simulink model "simu_acc"  (R2019b)
settings: Solver=VariableStepAuto  StartTime=0.0  StopTime=200.0  RelTol=1e-3
values from neighbouring files (symbols this model uses):
  d_0 = 150    [parametros.m]
  d_ref = 50    [parametros.m]
  delta_d_ref = 0    [parametros.m]
  delta_theta = 0    [parametros.m]
  delta_u_ref = 0    [parametros.m]
  delta_uw = 0    [parametros.m]
  delta_vl = -5    [parametros.m]
  K = 1/(rho*Cd*A*(V0 + VW0))    [modelo_lin.m]
  Kd_pos = 0    [parametros.m]
  Kd_vel = 0    [parametros.m]
  Ki_pos = 0    [parametros.m]
  Ki_vel = 5    [parametros.m]
  Kp_pos = 0.08    [parametros.m]
  Kp_vel = 100    [parametros.m]
  pend_vl = 1    [parametros.m]
  t_pert = 150    [parametros.m]
  t_ref = 20    [parametros.m]
  t_vl = 150    [parametros.m]
  tau = m/(rho*Cd*A*(V0 + VW0))    [modelo_lin.m]
  theta = in(3)    [dinamica.m]    (also in parametros.m = 0)
  u_ini = 20    [parametros.m]
  u_ref = 20    [parametros.m]
  uw = in(2)    [dinamica.m]    (also in parametros.m = 20)
  vl = 18    [parametros.m]
  wc_filt_vel = 5    [parametros.m]
libraries: simulink x6
settings Model: Creator=isidro  LastModifiedBy=isidro

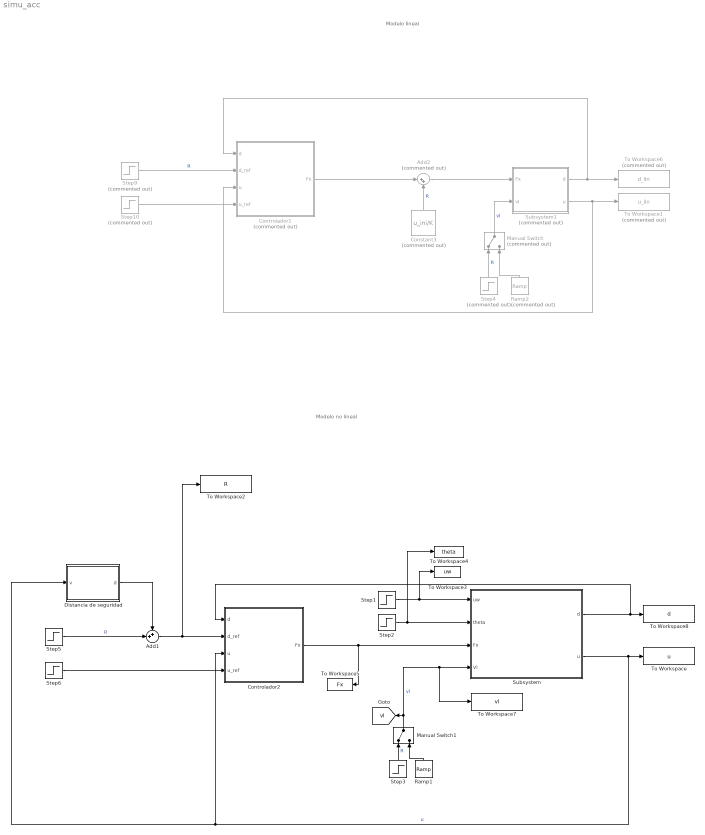
== system simu_acc ==
  note: Modelo no lineal
  note: Modelo lineal
  Add1 : Sum  Inputs=++|
  Add2 : Sum  Commented=on  Inputs=|++
  Constant3 : Constant  Commented=on  Value=u_ini/K  SampleTime=0
  Controlador1 : Subsystem  Commented=on
  Controlador2 : Subsystem
  Distancia de seguridad : Subsystem
  Manual Switch : ManualSwitch  Commented=on
  Manual Switch1 : ManualSwitch
  Ramp1 : simulink/Sources/Ramp  slope=pend_vl  start=t_vl  InitialOutput=vl
  Ramp2 : simulink/Sources/Ramp  Commented=on  slope=pend_vl  start=t_vl  InitialOutput=vl
  Step1 : Step  Time=t_pert  Before=uw  After=uw+delta_uw  SampleTime=0
  Step10 : Step  Commented=on  Time=t_ref  Before=u_ref  After=u_ref + delta_u_ref  SampleTime=0
  Step2 : Step  Time=t_pert  Before=theta  After=theta+delta_theta  SampleTime=0
  Step3 : Step  Time=t_vl  Before=vl  After=delta_vl+vl  SampleTime=0
  Step4 : Step  Commented=on  Time=t_vl  Before=vl  After=delta_vl+vl  SampleTime=0
  Step5 : Step  Time=t_ref  Before=d_ref  After=d_ref + delta_d_ref  SampleTime=0
  Step6 : Step  Time=t_ref  Before=u_ref  After=u_ref + delta_u_ref  SampleTime=0
  Step9 : Step  Commented=on  Time=t_ref  Before=d_ref  After=d_ref + delta_d_ref  SampleTime=0
  Subsystem : Subsystem
  Subsystem1 : Subsystem  Commented=on
  To Workspace : ToWorkspace  VariableName=u  SaveFormat=Timeseries  SampleTime=-1
  To Workspace1 : ToWorkspace  Commented=on  VariableName=u_lin  SaveFormat=Timeseries  SampleTime=-1
  To Workspace2 : ToWorkspace  VariableName=R  SaveFormat=Timeseries  SampleTime=-1
  To Workspace3 : ToWorkspace  VariableName=uw  SaveFormat=Timeseries  SampleTime=-1
  To Workspace4 : ToWorkspace  VariableName=theta  SaveFormat=Timeseries  SampleTime=-1
  To Workspace5 : ToWorkspace  VariableName=Fx  SaveFormat=Timeseries  SampleTime=-1
  To Workspace6 : ToWorkspace  Commented=on  VariableName=d_lin  SaveFormat=Timeseries  SampleTime=-1
  To Workspace7 : ToWorkspace  VariableName=vl  SaveFormat=Timeseries  SampleTime=-1
  To Workspace8 : ToWorkspace  VariableName=d  SaveFormat=Timeseries  SampleTime=-1
  tag scope: vl=global
  wires:
  Subsystem/2(u) -> Controlador2/3(u), Distancia de seguridad/1(v), To Workspace/1  "u"
  Step1/1 -> To Workspace3/1, Subsystem/1(uw)
  Step2/1 -> To Workspace4/1, Subsystem/2(theta)
  Step4/1 -> Manual Switch/1  "R"
  Ramp2/1 -> Manual Switch/2
  Manual Switch/1 -> Subsystem1/2(vl)  "vl"
  Subsystem1/2(u) -> Controlador1/3(u), To Workspace1/1
  Subsystem1/1(d) -> Controlador1/1(d), To Workspace6/1
  Manual Switch1/1 -> [vl], To Workspace7/1, Subsystem/4(Vl)  "vl"
  Ramp1/1 -> Manual Switch1/2
  Step3/1 -> Manual Switch1/1  "R"
  Subsystem/1(d) -> Controlador2/1(d), To Workspace8/1
  Constant3/1 -> Add2/2  "R"
  Add2/1 -> Subsystem1/1(Fx)
  Step6/1 -> Controlador2/4(u_ref)
  Controlador2/1(Fx) -> To Workspace5/1, Subsystem/3(Fx)
  Step10/1 -> Controlador1/4(u_ref)
  Controlador1/1(Fx) -> Add2/1
  Step9/1 -> Controlador1/2(d_ref)  "R"
  Distancia de seguridad/1(d) -> Add1/1
  Step5/1 -> Add1/2  "R"
  Add1/1 -> To Workspace2/1, Controlador2/2(d_ref)

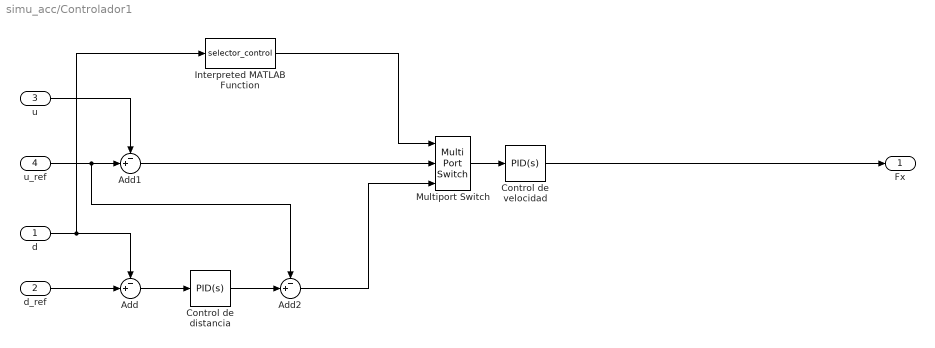
== system simu_acc/Controlador1 ==
  d : Inport
  d_ref : Inport  Port=2
  u : Inport  Port=3
  u_ref : Inport  Port=4
  Add : Sum  Inputs=-+|
  Add1 : Sum  Inputs=-+|
  Add2 : Sum  Inputs=-+|
  Control de distancia : simulink/Continuous/PID Controller  Controller=PID  Form=Parallel  TimeDomain=Continuous-time  SampleTime=-1  IntegratorMethod=Forward Euler  FilterMethod=Forward Euler  ControllerParametersSource=internal  P=Kp_pos  I=Ki_pos  D=Kd_pos  UseFilter=on  N=100  TunerSelectOption=Transfer Function Based (PID Tuner App)  InitialConditionSource=internal  InitialConditionForIntegrator=0  InitialConditionForFilter=0  DifferentiatorICPrevScaledInput=0  ExternalReset=none  TrackingMode=off  Kt=1  LimitOutput=off  UpperSaturationLimit=inf  LowerSaturationLimit=-inf  LinearizeAsGain=on  AntiWindupMode=none  Kb=1  POutMin=[]  POutMax=[]  IOutMin=[]  IOutMax=[]  DOutMin=[]  DOutMax=[]  NOutMin=[]  NOutMax=[]  SumOutMin=[]  SumOutMax=[]  SaturationOutMin=[]  SaturationOutMax=[]  PParamMin=[]  PParamMax=[]  IParamMin=[]  IParamMax=[]  DParamMin=[]  DParamMax=[]  NParamMin=[]  NParamMax=[]  KbParamMin=[]  KbParamMax=[]  KtParamMin=[]  KtParamMax=[]  KbOutMin=[]  KbOutMax=[]  KtOutMin=[]  KtOutMax=[]  IntegratorOutMin=[]  IntegratorOutMax=[]  FilterOutMin=[]  FilterOutMax=[]  SumI1OutMin=[]  SumI1OutMax=[]  SumI2OutMin=[]  SumI2OutMax=[]  SumI3OutMin=[]  SumI3OutMax=[]  SumI4OutMin=[]  SumI4OutMax=[]  SumDOutMin=[]  SumDOutMax=[]  DifferentiatorOutMin=[]  DifferentiatorOutMax=[]  FilterDiffOutCoefMin=[]  FilterDiffOutCoefMax=[]  ReciprocalOutMin=[]  ReciprocalOutMax=[]  SumDenOutMin=[]  SumDenOutMax=[]  SumNumOutMin=[]  SumNumOutMax=[]  DivideOutMin=[]  DivideOutMax=[]  IntegratorContinuousStateAttributes=''  IntegratorStateMustResolveToSignalObject=off  IntegratorRTWStateStorageClass=Auto  FilterContinuousStateAttributes=''  FilterStateMustResolveToSignalObject=off  FilterRTWStateStorageClass=Auto  ParallelPVariant=InternalParameters  IdealPVariant=Disabled  IVariant=InternalParameters  DVariant=InternalParameters  IntegratorVariant=Continuous  SatVariant=Disabled  AWVariant=Passthrough  PCopyVariant=Disabled  TRVariant=Disabled  FdbkBlocksVariant=Forward  IdealPFdbkVariant=Disabled  SatFdbkVariant=Disabled  DerivativeFilterVariant=ContFilter  NVariant=InternalParameters  NCopyVariant=Disabled  FilterICVariant=InternalICsFilter  IntegratorICVariant=InternalICs  ExternalResetVariant=Disabled  TRSumVariant=Passthrough  SumFdbkVariant=Disabled  SumVariant=Sum_PID
  Control de velocidad : simulink/Continuous/PID Controller  Controller=PID  Form=Parallel  TimeDomain=Continuous-time  SampleTime=-1  IntegratorMethod=Forward Euler  FilterMethod=Forward Euler  ControllerParametersSource=internal  P=Kp_vel  I=Ki_vel  D=Kd_vel  UseFilter=on  N=100  TunerSelectOption=Transfer Function Based (PID Tuner App)  InitialConditionSource=internal  InitialConditionForIntegrator=0  InitialConditionForFilter=0  DifferentiatorICPrevScaledInput=0  ExternalReset=none  TrackingMode=off  Kt=1  LimitOutput=off  UpperSaturationLimit=inf  LowerSaturationLimit=-inf  LinearizeAsGain=on  AntiWindupMode=none  Kb=1  POutMin=[]  POutMax=[]  IOutMin=[]  IOutMax=[]  DOutMin=[]  DOutMax=[]  NOutMin=[]  NOutMax=[]  SumOutMin=[]  SumOutMax=[]  SaturationOutMin=[]  SaturationOutMax=[]  PParamMin=[]  PParamMax=[]  IParamMin=[]  IParamMax=[]  DParamMin=[]  DParamMax=[]  NParamMin=[]  NParamMax=[]  KbParamMin=[]  KbParamMax=[]  KtParamMin=[]  KtParamMax=[]  KbOutMin=[]  KbOutMax=[]  KtOutMin=[]  KtOutMax=[]  IntegratorOutMin=[]  IntegratorOutMax=[]  FilterOutMin=[]  FilterOutMax=[]  SumI1OutMin=[]  SumI1OutMax=[]  SumI2OutMin=[]  SumI2OutMax=[]  SumI3OutMin=[]  SumI3OutMax=[]  SumI4OutMin=[]  SumI4OutMax=[]  SumDOutMin=[]  SumDOutMax=[]  DifferentiatorOutMin=[]  DifferentiatorOutMax=[]  FilterDiffOutCoefMin=[]  FilterDiffOutCoefMax=[]  ReciprocalOutMin=[]  ReciprocalOutMax=[]  SumDenOutMin=[]  SumDenOutMax=[]  SumNumOutMin=[]  SumNumOutMax=[]  DivideOutMin=[]  DivideOutMax=[]  IntegratorContinuousStateAttributes=''  IntegratorStateMustResolveToSignalObject=off  IntegratorRTWStateStorageClass=Auto  FilterContinuousStateAttributes=''  FilterStateMustResolveToSignalObject=off  FilterRTWStateStorageClass=Auto  ParallelPVariant=InternalParameters  IdealPVariant=Disabled  IVariant=InternalParameters  DVariant=InternalParameters  IntegratorVariant=Continuous  SatVariant=Disabled  AWVariant=Passthrough  PCopyVariant=Disabled  TRVariant=Disabled  FdbkBlocksVariant=Forward  IdealPFdbkVariant=Disabled  SatFdbkVariant=Disabled  DerivativeFilterVariant=ContFilter  NVariant=InternalParameters  NCopyVariant=Disabled  FilterICVariant=InternalICsFilter  IntegratorICVariant=InternalICs  ExternalResetVariant=Disabled  TRSumVariant=Passthrough  SumFdbkVariant=Disabled  SumVariant=Sum_PID
  Interpreted MATLAB Function : MATLABFcn  MATLABFcn=selector_control
  Multiport Switch : MultiPortSwitch  Inputs=2
  Fx : Outport
  wires:
  d/1 -> Add/1, Interpreted MATLAB Function/1
  d_ref/1 -> Add/2
  u_ref/1 -> Add2/1, Add1/2
  u/1 -> Add1/1
  Add/1 -> Control de distancia/1
  Multiport Switch/1 -> Control de velocidad/1
  Control de distancia/1 -> Add2/2
  Add1/1 -> Multiport Switch/2
  Add2/1 -> Multiport Switch/3
  Interpreted MATLAB Function/1 -> Multiport Switch/1
  Control de velocidad/1 -> Fx/1

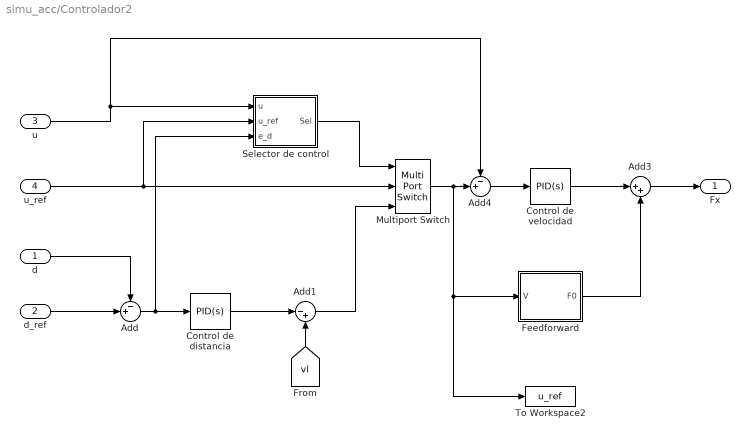
== system simu_acc/Controlador2 ==
  d : Inport
  d_ref : Inport  Port=2
  u : Inport  Port=3
  u_ref : Inport  Port=4
  Add : Sum  Inputs=-+|
  Add1 : Sum  Inputs=|-+
  Add3 : Sum  Inputs=|++
  Add4 : Sum  Inputs=-+|
  Control de distancia : simulink/Continuous/PID Controller  Controller=PID  Form=Parallel  TimeDomain=Continuous-time  SampleTime=-1  IntegratorMethod=Forward Euler  FilterMethod=Forward Euler  ControllerParametersSource=internal  P=Kp_pos  I=Ki_pos  D=Kd_pos  UseFilter=on  N=100  TunerSelectOption=Transfer Function Based (PID Tuner App)  InitialConditionSource=internal  InitialConditionForIntegrator=0  InitialConditionForFilter=0  DifferentiatorICPrevScaledInput=0  ExternalReset=none  TrackingMode=off  Kt=1  LimitOutput=off  UpperSaturationLimit=inf  LowerSaturationLimit=-inf  LinearizeAsGain=on  AntiWindupMode=none  Kb=1  POutMin=[]  POutMax=[]  IOutMin=[]  IOutMax=[]  DOutMin=[]  DOutMax=[]  NOutMin=[]  NOutMax=[]  SumOutMin=[]  SumOutMax=[]  SaturationOutMin=[]  SaturationOutMax=[]  PParamMin=[]  PParamMax=[]  IParamMin=[]  IParamMax=[]  DParamMin=[]  DParamMax=[]  NParamMin=[]  NParamMax=[]  KbParamMin=[]  KbParamMax=[]  KtParamMin=[]  KtParamMax=[]  KbOutMin=[]  KbOutMax=[]  KtOutMin=[]  KtOutMax=[]  IntegratorOutMin=[]  IntegratorOutMax=[]  FilterOutMin=[]  FilterOutMax=[]  SumI1OutMin=[]  SumI1OutMax=[]  SumI2OutMin=[]  SumI2OutMax=[]  SumI3OutMin=[]  SumI3OutMax=[]  SumI4OutMin=[]  SumI4OutMax=[]  SumDOutMin=[]  SumDOutMax=[]  DifferentiatorOutMin=[]  DifferentiatorOutMax=[]  FilterDiffOutCoefMin=[]  FilterDiffOutCoefMax=[]  ReciprocalOutMin=[]  ReciprocalOutMax=[]  SumDenOutMin=[]  SumDenOutMax=[]  SumNumOutMin=[]  SumNumOutMax=[]  DivideOutMin=[]  DivideOutMax=[]  IntegratorContinuousStateAttributes=''  IntegratorStateMustResolveToSignalObject=off  IntegratorRTWStateStorageClass=Auto  FilterContinuousStateAttributes=''  FilterStateMustResolveToSignalObject=off  FilterRTWStateStorageClass=Auto  ParallelPVariant=InternalParameters  IdealPVariant=Disabled  IVariant=InternalParameters  DVariant=InternalParameters  IntegratorVariant=Continuous  SatVariant=Disabled  AWVariant=Passthrough  PCopyVariant=Disabled  TRVariant=Disabled  FdbkBlocksVariant=Forward  IdealPFdbkVariant=Disabled  SatFdbkVariant=Disabled  DerivativeFilterVariant=ContFilter  NVariant=InternalParameters  NCopyVariant=Disabled  FilterICVariant=InternalICsFilter  IntegratorICVariant=InternalICs  ExternalResetVariant=Disabled  TRSumVariant=Passthrough  SumFdbkVariant=Disabled  SumVariant=Sum_PID
  Control de velocidad : simulink/Continuous/PID Controller  Controller=PID  Form=Parallel  TimeDomain=Continuous-time  SampleTime=-1  IntegratorMethod=Forward Euler  FilterMethod=Forward Euler  ControllerParametersSource=internal  P=Kp_vel  I=Ki_vel  D=Kd_vel  UseFilter=on  N=wc_filt_vel  TunerSelectOption=Transfer Function Based (PID Tuner App)  InitialConditionSource=internal  InitialConditionForIntegrator=0  InitialConditionForFilter=0  DifferentiatorICPrevScaledInput=0  ExternalReset=none  TrackingMode=off  Kt=1  LimitOutput=off  UpperSaturationLimit=inf  LowerSaturationLimit=-inf  LinearizeAsGain=on  AntiWindupMode=none  Kb=1  POutMin=[]  POutMax=[]  IOutMin=[]  IOutMax=[]  DOutMin=[]  DOutMax=[]  NOutMin=[]  NOutMax=[]  SumOutMin=[]  SumOutMax=[]  SaturationOutMin=[]  SaturationOutMax=[]  PParamMin=[]  PParamMax=[]  IParamMin=[]  IParamMax=[]  DParamMin=[]  DParamMax=[]  NParamMin=[]  NParamMax=[]  KbParamMin=[]  KbParamMax=[]  KtParamMin=[]  KtParamMax=[]  KbOutMin=[]  KbOutMax=[]  KtOutMin=[]  KtOutMax=[]  IntegratorOutMin=[]  IntegratorOutMax=[]  FilterOutMin=[]  FilterOutMax=[]  SumI1OutMin=[]  SumI1OutMax=[]  SumI2OutMin=[]  SumI2OutMax=[]  SumI3OutMin=[]  SumI3OutMax=[]  SumI4OutMin=[]  SumI4OutMax=[]  SumDOutMin=[]  SumDOutMax=[]  DifferentiatorOutMin=[]  DifferentiatorOutMax=[]  FilterDiffOutCoefMin=[]  FilterDiffOutCoefMax=[]  ReciprocalOutMin=[]  ReciprocalOutMax=[]  SumDenOutMin=[]  SumDenOutMax=[]  SumNumOutMin=[]  SumNumOutMax=[]  DivideOutMin=[]  DivideOutMax=[]  IntegratorContinuousStateAttributes=''  IntegratorStateMustResolveToSignalObject=off  IntegratorRTWStateStorageClass=Auto  FilterContinuousStateAttributes=''  FilterStateMustResolveToSignalObject=off  FilterRTWStateStorageClass=Auto  ParallelPVariant=InternalParameters  IdealPVariant=Disabled  IVariant=InternalParameters  DVariant=InternalParameters  IntegratorVariant=Continuous  SatVariant=Disabled  AWVariant=Passthrough  PCopyVariant=Disabled  TRVariant=Disabled  FdbkBlocksVariant=Forward  IdealPFdbkVariant=Disabled  SatFdbkVariant=Disabled  DerivativeFilterVariant=ContFilter  NVariant=InternalParameters  NCopyVariant=Disabled  FilterICVariant=InternalICsFilter  IntegratorICVariant=InternalICs  ExternalResetVariant=Disabled  TRSumVariant=Passthrough  SumFdbkVariant=Disabled  SumVariant=Sum_PID
  Feedforward : Subsystem
  Multiport Switch : MultiPortSwitch  Inputs=2
  Selector de control : Subsystem
  To Workspace2 : ToWorkspace  VariableName=u_ref  SaveFormat=Timeseries  SampleTime=-1
  Fx : Outport
  wires:
  d/1 -> Add/1
  d_ref/1 -> Add/2
  Add3/1 -> Fx/1
  Control de velocidad/1 -> Add3/1
  Multiport Switch/1 -> Feedforward/1(V), To Workspace2/1, Add4/2
  u/1 -> Selector de control/1(u), Add4/1
  u_ref/1 -> Selector de control/2(u_ref), Multiport Switch/2
  Add4/1 -> Control de velocidad/1
  Control de distancia/1 -> Add1/1
  Add1/1 -> Multiport Switch/3
  Add/1 -> Selector de control/3(e_d), Control de distancia/1
  Feedforward/1(F0) -> Add3/2
  [vl] -> Add1/2
  Selector de control/1(Sel) -> Multiport Switch/1

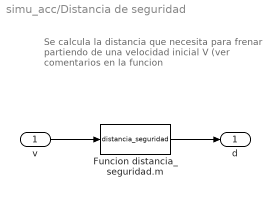
== system simu_acc/Distancia de seguridad ==
  note: Se calcula la distancia que necesita para frenar partiendo de una velocidad inicial V (ver comentarios en la funcion
  v : Inport
  Funcion distancia_seguridad.m : MATLABFcn  MATLABFcn=distancia_seguridad
  d : Outport
  wires:
  Funcion distancia_seguridad.m/1 -> d/1
  v/1 -> Funcion distancia_seguridad.m/1

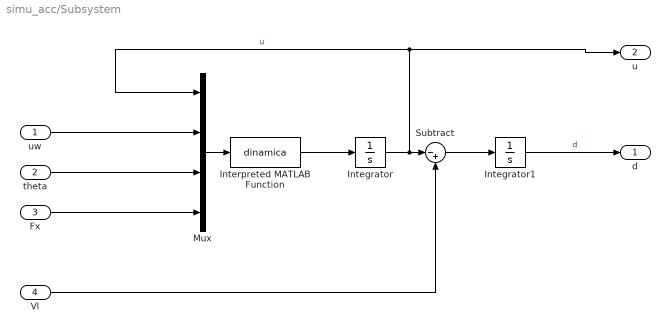
== system simu_acc/Subsystem ==
  uw : Inport
  theta : Inport  Port=2
  Fx : Inport  Port=3
  Vl : Inport  Port=4
  Integrator : Integrator  InitialCondition=u_ini
  Integrator1 : Integrator  InitialCondition=d_0
  Interpreted MATLAB Function : MATLABFcn  MATLABFcn=dinamica
  Mux : Mux
  Subtract : Sum  Inputs=|-+
  d : Outport
  u : Outport  Port=2
  wires:
  Interpreted MATLAB Function/1 -> Integrator/1
  Mux/1 -> Interpreted MATLAB Function/1
  Fx/1 -> Mux/4
  theta/1 -> Mux/3
  Integrator/1 -> Subtract/1, Mux/1, u/1  "u"
  uw/1 -> Mux/2
  Vl/1 -> Subtract/2
  Subtract/1 -> Integrator1/1
  Integrator1/1 -> d/1  "d"

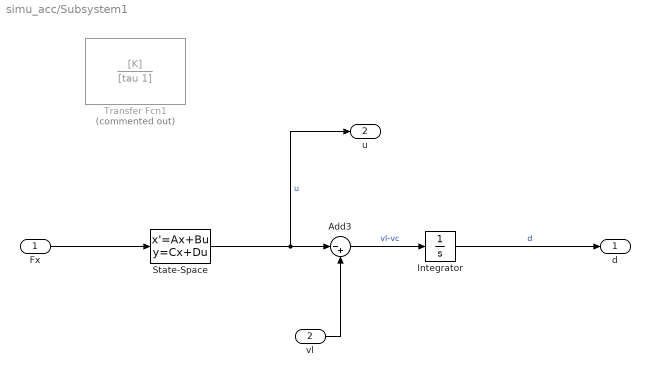
== system simu_acc/Subsystem1 ==
  Fx : Inport
  vl : Inport  Port=2
  Add3 : Sum  Inputs=|-+
  Integrator : Integrator  InitialCondition=d_0
  State-Space : StateSpace  A=-1/tau  B=K/tau  D=0  InitialCondition=u_ini
  Transfer Fcn1 : TransferFcn  Commented=on  Numerator=[K]  Denominator=[tau 1]
  d : Outport
  u : Outport  Port=2
  wires:
  Fx/1 -> State-Space/1
  vl/1 -> Add3/2
  Add3/1 -> Integrator/1  "vl-vc"
  State-Space/1 -> u/1, Add3/1  "u"
  Integrator/1 -> d/1  "d"

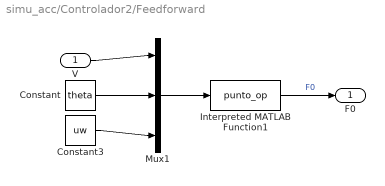
== system simu_acc/Controlador2/Feedforward ==
  V : Inport
  Constant : Constant  Value=theta
  Constant3 : Constant  Value=uw
  Interpreted MATLAB Function1 : MATLABFcn  MATLABFcn=punto_op  OutputDimensions=1
  Mux1 : Mux  Inputs=3
  F0 : Outport
  wires:
  V/1 -> Mux1/1
  Interpreted MATLAB Function1/1 -> F0/1  "F0"
  Constant/1 -> Mux1/2
  Constant3/1 -> Mux1/3
  Mux1/1 -> Interpreted MATLAB Function1/1

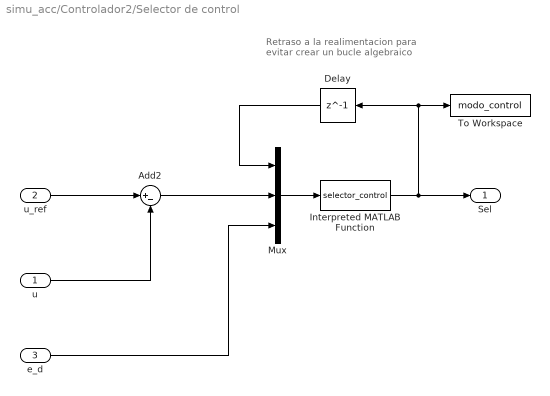
== system simu_acc/Controlador2/Selector de control ==
  note: Retraso a la realimentacion para
      | evitar crear un bucle algebraico
  u : Inport
  u_ref : Inport  Port=2
  e_d : Inport  Port=3
  Add2 : Sum  Inputs=|+-
  Delay : Delay  DelayLength=1
  Interpreted MATLAB Function : MATLABFcn  MATLABFcn=selector_control  OutputDimensions=1
  Mux : Mux  Inputs=3
  To Workspace : ToWorkspace  VariableName=modo_control  SaveFormat=Timeseries  SampleTime=-1
  Sel : Outport
  wires:
  u/1 -> Add2/2
  Interpreted MATLAB Function/1 -> Delay/1, To Workspace/1, Sel/1
  e_d/1 -> Mux/3
  Add2/1 -> Mux/2
  Delay/1 -> Mux/1
  u_ref/1 -> Add2/1
  Mux/1 -> Interpreted MATLAB Function/1
